simulink model "ieee_80211n"  (Simulink 7.4)
settings: Solver=ode45  StartTime=0.0  StopTime=2.076*100  RelTol=1e-3
PreLoadFcn:
  | EbNo = 1; maxNumErrs = 100; maxNumBits = 1e6;
undefined symbols (not defined in the file or in its folder): bchgenpoly
libraries: dspindex x11, dspbuff3 x6, commblkintrlv2 x4, dspxfrm3 x4, commdigbbndam3 x4, commblkcod2 x2, commsequence2 x2, commchan3 x1, commsink2 x1, commrandsrc2 x1
settings Model: Creator=nick  LastModifiedBy=nick

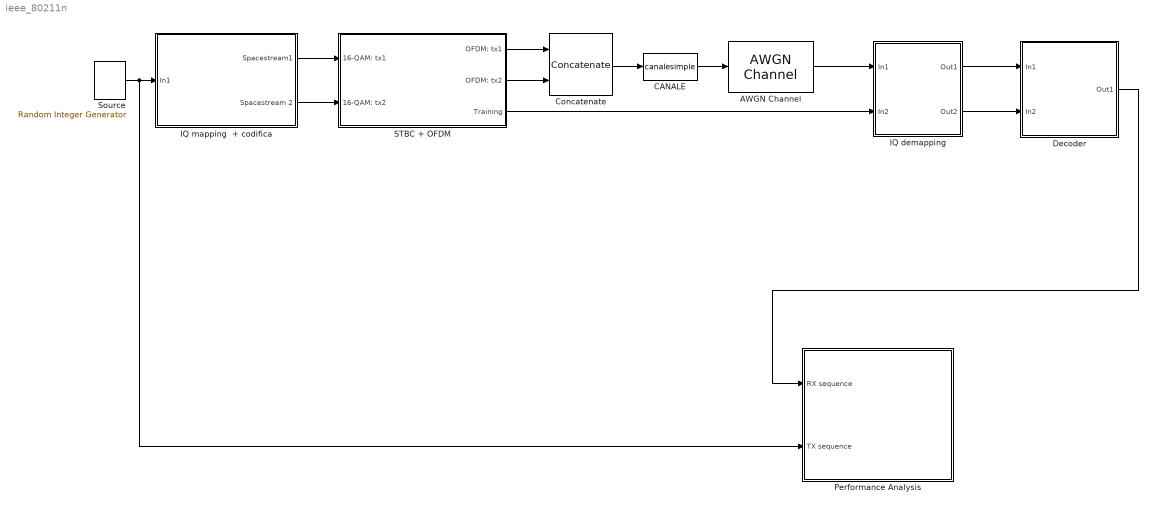
== system ieee_80211n ==
  AWGN Channel : commchan3/AWGN Channel  SystemSampleTime=-1  seed=67  noiseMode="Signal to noise ratio  (SNR)"  EbNodB=EbNo  EsNodB=10  SNRdB=SNR  bitsPerSym=264  Ps=1  Tsym=0.416  variance=1
  CANALE : MATLABFcn  MATLABFcn=canalesimple  Output1D=off
  Concatenate : Concatenate  Mode=Multidimensional array  ConcatenateDimension=2
  Decoder : Subsystem
  IQ demapping : Subsystem
  IQ mapping  + codifica : Subsystem
  Performance Analysis : Subsystem
  STBC + OFDM : Subsystem
  Source : commrandsrc2/Random Integer Generator  SystemSampleTime=-1  mul=2  seed=37  Ts=2e-3  frameBased=on  sampPerFrame=4  orient=off  outDataType=boolean
  wires:
  IQ mapping  + codifica/2(Spacestream 2) -> STBC + OFDM/2(16-QAM: tx2)
  IQ mapping  + codifica/1(Spacestream1) -> STBC + OFDM/1(16-QAM: tx1)
  Concatenate/1 -> CANALE/1
  Source/1 -> IQ mapping  + codifica/1(In1), Performance Analysis/2(TX sequence)
  STBC + OFDM/1(OFDM: tx1) -> Concatenate/1
  STBC + OFDM/2(OFDM: tx2) -> Concatenate/2
  STBC + OFDM/3(Training) -> IQ demapping/2(In2)
  CANALE/1 -> AWGN Channel/1
  IQ demapping/1(Out1) -> Decoder/1(In1)
  IQ demapping/2(Out2) -> Decoder/2(In2)
  Decoder/1(Out1) -> Performance Analysis/1(RX sequence)
  AWGN Channel/1 -> IQ demapping/1(In1)

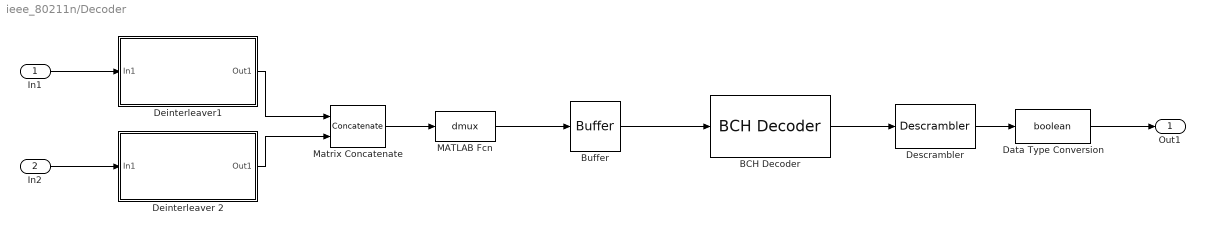
== system ieee_80211n/Decoder ==
  In1 : Inport
  In2 : Inport  Port=2
  BCH Decoder : commblkcod2/BCH Decoder  n=8  k=4  specPrimPoly=off  prPoly=de2bi(primpoly(4, 'nodisplay'), 'left-msb')  specGenPoly=off  genPoly=bchgenpoly(15,5)  specDisableGenCheck=off  specPuncture=off  punctVec=[ones(8,1); zeros(2,1)]  specErasurePort=off  showNumErr=off
  Buffer : dspbuff3/Buffer  N=8  V=0  ic=0
  Data Type Conversion : DataTypeConversion  OutDataTypeMode=boolean  OutDataType=fixdt(1, 16)  OutScaling=2^0  OutDataTypeStr=boolean
  Deinterleaver 2 : Subsystem
  Deinterleaver1 : Subsystem
  Descrambler : commsequence2/Descrambler  M=2  poly=[1 0 0 1 0 0 0 1]  ini_sta=[0 0 0 0 0 0 1]
  MATLAB Fcn : MATLABFcn  MATLABFcn=dmux  Output1D=off
  Matrix Concatenate : Concatenate  Mode=Multidimensional array  ConcatenateDimension=2
  Out1 : Outport
  wires:
  In1/1 -> Deinterleaver1/1(In1)
  In2/1 -> Deinterleaver 2/1(In1)
  Matrix Concatenate/1 -> MATLAB Fcn/1
  Deinterleaver 2/1(Out1) -> Matrix Concatenate/2
  Deinterleaver1/1(Out1) -> Matrix Concatenate/1
  BCH Decoder/1 -> Descrambler/1
  MATLAB Fcn/1 -> Buffer/1
  Data Type Conversion/1 -> Out1/1
  Descrambler/1 -> Data Type Conversion/1
  Buffer/1 -> BCH Decoder/1

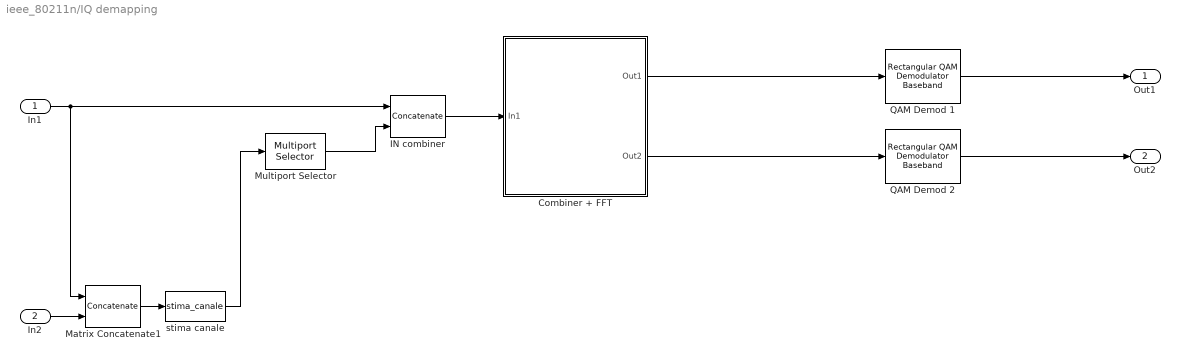
== system ieee_80211n/IQ demapping ==
  In1 : Inport
  In2 : Inport  Port=2
  Combiner + FFT : Subsystem
  IN combiner : Concatenate  Mode=Multidimensional array
  Matrix Concatenate1 : Concatenate  Mode=Multidimensional array  ConcatenateDimension=2
  Multiport Selector : dspindex/Multiport Selector  rowsOrCols=Columns  idxCellArray={ 1:2 }  idxErrMode=Clip Index
  QAM Demod 1 : commdigbbndam3/Rectangular QAM Demodulator Baseband  DialogController=commDDGCreate  DialogControllerArgs=DataTag2  M=16  PowType=Average Power  MinDist=2  AvgPow=5.25  PeakPow=1  Ph=0  Dec=Gray  Mapping=[0:15]  OutType=Bit  DecType=Hard decision  VarSource=Port  Variance=1  outDtype1=Inherit via internal rule  outDtype2=Inherit via internal rule  derotateFactorWordLen=16  denormFactorWordLen=16  prodOutWordLen=32  prodOutRoundingMode=Floor  prodOutOverflowMode=Wrap  sumWordLen=32
  QAM Demod 2 : commdigbbndam3/Rectangular QAM Demodulator Baseband  DialogController=commDDGCreate  DialogControllerArgs=DataTag3  M=16  PowType=Average Power  MinDist=2  AvgPow=5.25  PeakPow=1  Ph=0  Dec=Gray  Mapping=[0:15]  OutType=Bit  DecType=Hard decision  VarSource=Port  Variance=1  outDtype1=Inherit via internal rule  outDtype2=Inherit via internal rule  derotateFactorWordLen=16  denormFactorWordLen=16  prodOutWordLen=32  prodOutRoundingMode=Floor  prodOutOverflowMode=Wrap  sumWordLen=32
  stima canale : MATLABFcn  MATLABFcn=stima_canale  Output1D=off
  Out1 : Outport
  Out2 : Outport  Port=2
  wires:
  In1/1 -> Matrix Concatenate1/1, IN combiner/1
  Matrix Concatenate1/1 -> stima canale/1
  IN combiner/1 -> Combiner + FFT/1(In1)
  stima canale/1 -> Multiport Selector/1
  Multiport Selector/1 -> IN combiner/2
  Combiner + FFT/1(Out1) -> QAM Demod 1/1
  Combiner + FFT/2(Out2) -> QAM Demod 2/1
  QAM Demod 1/1 -> Out1/1
  QAM Demod 2/1 -> Out2/1
  In2/1 -> Matrix Concatenate1/2

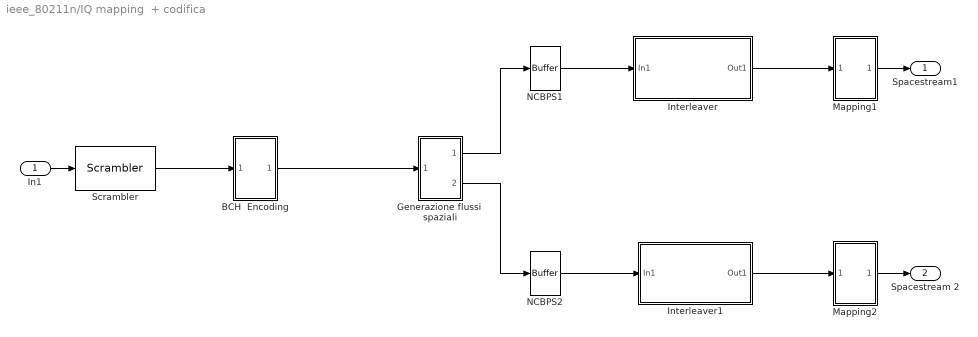
== system ieee_80211n/IQ mapping  + codifica ==
  In1 : Inport
  BCH  Encoding : Subsystem
  Generazione flussi  spaziali : Subsystem
  Interleaver : Subsystem  TreatAsAtomicUnit=on
  Interleaver1 : Subsystem  TreatAsAtomicUnit=on
  Mapping1 : Subsystem
  Mapping2 : Subsystem
  NCBPS1 : dspbuff3/Buffer  N=208  V=0  ic=0
  NCBPS2 : dspbuff3/Buffer  N=208  V=0  ic=0
  Scrambler : commsequence2/Scrambler  M=2  poly=[1 0 0 1 0 0 0 1]  ini_sta=[0 0 0 0 0 0 1]
  Spacestream1 : Outport
  Spacestream 2 : Outport  Port=2
  wires:
  Scrambler/1 -> BCH  Encoding/1(In1)
  Generazione flussi  spaziali/2(Out2) -> NCBPS2/1
  NCBPS1/1 -> Interleaver/1(In1)
  NCBPS2/1 -> Interleaver1/1(In1)
  Generazione flussi  spaziali/1(Out1) -> NCBPS1/1
  Interleaver1/1(Out1) -> Mapping2/1(In1)
  Interleaver/1(Out1) -> Mapping1/1(In1)
  Mapping1/1(Out1) -> Spacestream1/1
  Mapping2/1(Out1) -> Spacestream 2/1
  In1/1 -> Scrambler/1
  BCH  Encoding/1(Out1) -> Generazione flussi  spaziali/1(In1)

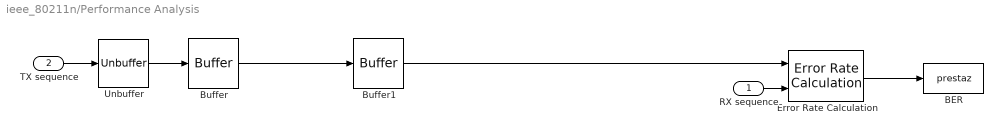
== system ieee_80211n/Performance Analysis ==
  RX sequence : Inport
  TX sequence : Inport  Port=2
  BER : ToWorkspace  VariableName=prestaz  SampleTime=-1  SaveFormat=Array
      settings: MaxDataPoints=1
  Buffer : dspbuff3/Buffer  N=208  V=0  ic=0
  Buffer1 : dspbuff3/Buffer  N=4  V=0  ic=0
  Error Rate Calculation : commsink2/Error Rate Calculation  N=0  st_delay=0  cp_mode=Entire frame  subframe=[]  PMode=Port  WsName=ErrorVec  RsMode2=off  stop=off  numErr=maxNumErrs  maxBits=maxNumBits
  Unbuffer : dspbuff3/Unbuffer  ic=0
  wires:
  Unbuffer/1 -> Buffer/1
  Buffer/1 -> Buffer1/1
  Buffer1/1 -> Error Rate Calculation/1
  Error Rate Calculation/1 -> BER/1
  TX sequence/1 -> Unbuffer/1
  RX sequence/1 -> Error Rate Calculation/2

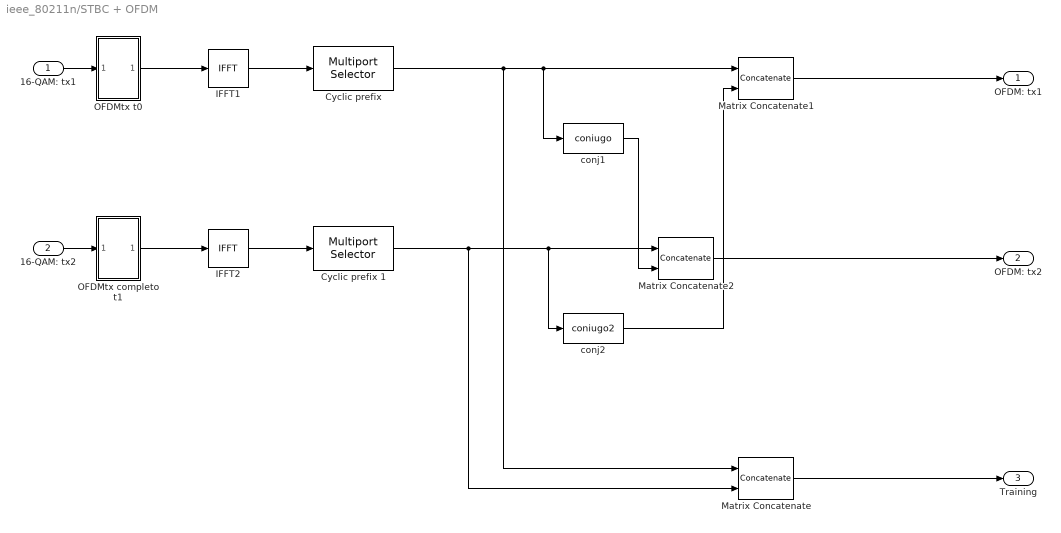
== system ieee_80211n/STBC + OFDM ==
  16-QAM: tx1 : Inport
  16-QAM: tx2 : Inport  Port=2
  Cyclic prefix : dspindex/Multiport Selector  rowsOrCols=Rows  idxCellArray={[1:64 2 1]'}  idxErrMode=Clip Index
  Cyclic prefix 1 : dspindex/Multiport Selector  rowsOrCols=Rows  idxCellArray={[1:64 2 1]'}  idxErrMode=Clip Index
  IFFT1 : dspxfrm3/IFFT  DialogController=dspDDGCreate  DialogControllerArgs=DataTag6  CompMethod=Table lookup  TableOpt=NEW  TableOptActive=Speed  BitRevOrder=off  cs_in=off  SkipNorm=on  InheritFFTLength=on  FFTLength=64  mode=Complex  outSamplingMode=Frame based  roundingMode=Floor  overflowMode=off
  IFFT2 : dspxfrm3/IFFT  DialogController=dspDDGCreate  DialogControllerArgs=DataTag7  CompMethod=Table lookup  TableOpt=NEW  TableOptActive=Speed  BitRevOrder=off  cs_in=off  SkipNorm=on  InheritFFTLength=on  FFTLength=64  mode=Complex  outSamplingMode=Frame based  roundingMode=Floor  overflowMode=off
  Matrix Concatenate : Concatenate  Mode=Multidimensional array
  Matrix Concatenate1 : Concatenate  Mode=Multidimensional array
  Matrix Concatenate2 : Concatenate  Mode=Multidimensional array
  OFDMtx completo t1 : Subsystem
  OFDMtx t0 : Subsystem
  conj1 : MATLABFcn  MATLABFcn=coniugo  Output1D=off
  conj2 : MATLABFcn  MATLABFcn=coniugo2  Output1D=off
  OFDM: tx1 : Outport  OutDataType=fixdt(1, 16)  OutScaling=2^0
  OFDM: tx2 : Outport  Port=2  OutDataType=fixdt(1, 16)  OutScaling=2^0
  Training : Outport  Port=3  OutDataType=fixdt(1, 16)  OutScaling=2^0
  wires:
  OFDMtx t0/1(Out1) -> IFFT1/1
  OFDMtx completo t1/1(Out1) -> IFFT2/1
  16-QAM: tx1/1 -> OFDMtx t0/1(In1)
  16-QAM: tx2/1 -> OFDMtx completo t1/1(In1)
  IFFT1/1 -> Cyclic prefix/1
  IFFT2/1 -> Cyclic prefix 1/1
  Cyclic prefix 1/1 -> Matrix Concatenate/2, conj2/1, Matrix Concatenate2/1
  Matrix Concatenate/1 -> Training/1
  Cyclic prefix/1 -> Matrix Concatenate1/1, conj1/1, Matrix Concatenate/1
  Matrix Concatenate1/1 -> OFDM: tx1/1
  conj1/1 -> Matrix Concatenate2/2
  Matrix Concatenate2/1 -> OFDM: tx2/1
  conj2/1 -> Matrix Concatenate1/2

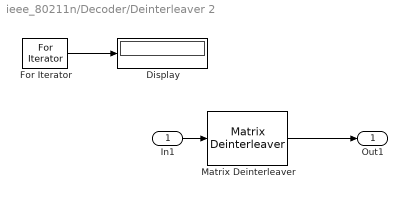
== system ieee_80211n/Decoder/Deinterleaver 2 ==
  In1 : Inport
  Display : Display
  For Iterator : ForIterator  IterationLimit=11
  Matrix Deinterleaver : commblkintrlv2/Matrix Deinterleaver  SystemSampleTime=-1  Nrows=16  Ncols=13
  Out1 : Outport  OutDataType=fixdt(1, 16)  OutScaling=2^0
  wires:
  In1/1 -> Matrix Deinterleaver/1
  Matrix Deinterleaver/1 -> Out1/1
  For Iterator/1 -> Display/1

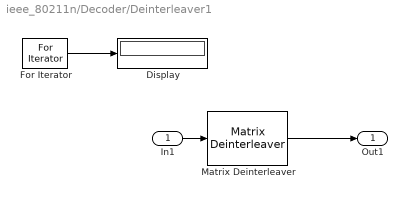
== system ieee_80211n/Decoder/Deinterleaver1 ==
  In1 : Inport
  Display : Display
  For Iterator : ForIterator  IterationLimit=11
  Matrix Deinterleaver : commblkintrlv2/Matrix Deinterleaver  SystemSampleTime=-1  Nrows=16  Ncols=13
  Out1 : Outport  OutDataType=fixdt(1, 16)  OutScaling=2^0
  wires:
  In1/1 -> Matrix Deinterleaver/1
  Matrix Deinterleaver/1 -> Out1/1
  For Iterator/1 -> Display/1

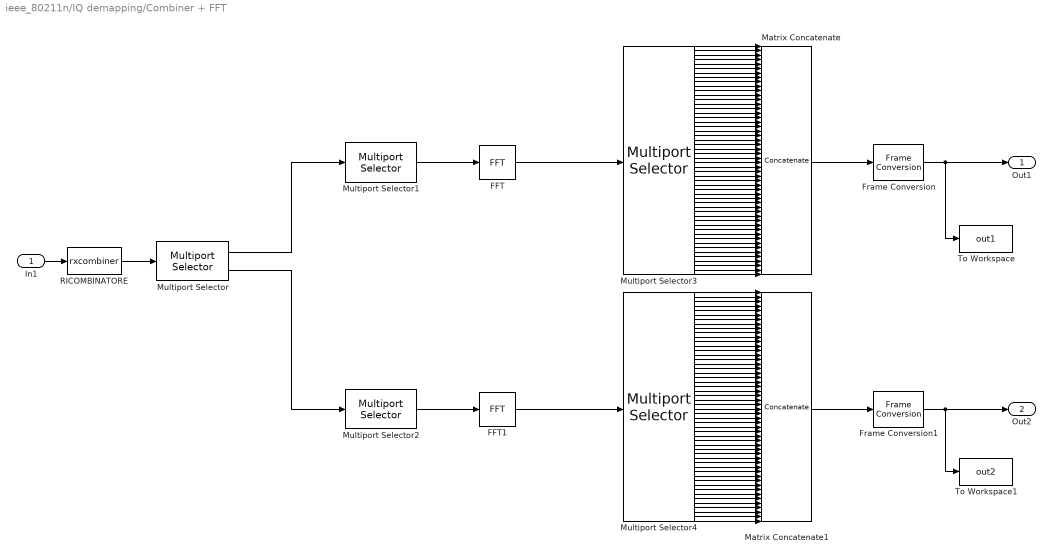
== system ieee_80211n/IQ demapping/Combiner + FFT ==
  In1 : Inport
  FFT : dspxfrm3/FFT  DialogController=dspDDGCreate  DialogControllerArgs=DataTag0  CompMethod=Table lookup  TableOpt=NEW  TableOptActive=Speed  BitRevOrder=off  InheritFFTLength=on  FFTLength=64  SkipNorm=off  roundingMode=Floor  overflowMode=off
  FFT1 : dspxfrm3/FFT  DialogController=dspDDGCreate  DialogControllerArgs=DataTag1  CompMethod=Table lookup  TableOpt=NEW  TableOptActive=Speed  BitRevOrder=off  InheritFFTLength=on  FFTLength=64  SkipNorm=off  roundingMode=Floor  overflowMode=off
  Frame Conversion : FrameConversion
  Frame Conversion1 : FrameConversion
  Matrix Concatenate : Concatenate  NumInputs=52  Mode=Multidimensional array
  Matrix Concatenate1 : Concatenate  NumInputs=52  Mode=Multidimensional array
  Multiport Selector : dspindex/Multiport Selector  rowsOrCols=Rows  idxCellArray={ [1:66],[67:132] }  idxErrMode=Clip Index
  Multiport Selector1 : dspindex/Multiport Selector  rowsOrCols=Rows  idxCellArray={ [1:64] }  idxErrMode=Clip Index
  Multiport Selector2 : dspindex/Multiport Selector  rowsOrCols=Rows  idxCellArray={ [1:64] }  idxErrMode=Clip Index
  Multiport Selector3 : dspindex/Multiport Selector  rowsOrCols=Rows  idxCellArray={2,3,4,5,6,7,9,10,11,12,13,14,15,16,17,18,19,20,21,23,24,25,26,27,28,29,37,38,39,40,41,42,44,45,46,47,48,49,50,51,52,53,54,55,56,58,59,60,61,62,63,64 }  idxErrMode=Clip Index
  Multiport Selector4 : dspindex/Multiport Selector  rowsOrCols=Rows  idxCellArray={2,3,4,5,6,7,9,10,11,12,13,14,15,16,17,18,19,20,21,23,24,25,26,27,28,29,37,38,39,40,41,42,44,45,46,47,48,49,50,51,52,53,54,55,56,58,59,60,61,62,63,64 }  idxErrMode=Clip Index
  RICOMBINATORE : MATLABFcn  MATLABFcn=rxcombiner  Output1D=off
  To Workspace : ToWorkspace  VariableName=out1  SampleTime=-1  SaveFormat=Array
  To Workspace1 : ToWorkspace  VariableName=out2  SampleTime=-1  SaveFormat=Array
  Out1 : Outport
  Out2 : Outport  Port=2
  wires:
  RICOMBINATORE/1 -> Multiport Selector/1
  Multiport Selector/1 -> Multiport Selector1/1
  Multiport Selector/2 -> Multiport Selector2/1
  Multiport Selector1/1 -> FFT/1
  Multiport Selector2/1 -> FFT1/1
  In1/1 -> RICOMBINATORE/1
  Frame Conversion/1 -> Out1/1, To Workspace/1
  FFT/1 -> Multiport Selector3/1
  Multiport Selector3/1 -> Matrix Concatenate/1
  Multiport Selector3/2 -> Matrix Concatenate/2
  Multiport Selector3/3 -> Matrix Concatenate/3
  Multiport Selector3/4 -> Matrix Concatenate/4
  Multiport Selector3/5 -> Matrix Concatenate/5
  Multiport Selector3/6 -> Matrix Concatenate/6
  Multiport Selector3/7 -> Matrix Concatenate/7
  Multiport Selector3/8 -> Matrix Concatenate/8
  Multiport Selector3/9 -> Matrix Concatenate/9
  Multiport Selector3/10 -> Matrix Concatenate/10
  Multiport Selector3/11 -> Matrix Concatenate/11
  Multiport Selector3/12 -> Matrix Concatenate/12
  Multiport Selector3/13 -> Matrix Concatenate/13
  Multiport Selector3/14 -> Matrix Concatenate/14
  Multiport Selector3/15 -> Matrix Concatenate/15
  Multiport Selector3/16 -> Matrix Concatenate/16
  Multiport Selector3/17 -> Matrix Concatenate/17
  Multiport Selector3/18 -> Matrix Concatenate/18
  Multiport Selector3/19 -> Matrix Concatenate/19
  Multiport Selector3/20 -> Matrix Concatenate/20
  Multiport Selector3/21 -> Matrix Concatenate/21
  Multiport Selector3/22 -> Matrix Concatenate/22
  Multiport Selector3/23 -> Matrix Concatenate/23
  Multiport Selector3/24 -> Matrix Concatenate/24
  Multiport Selector3/25 -> Matrix Concatenate/25
  Multiport Selector3/26 -> Matrix Concatenate/26
  Multiport Selector3/27 -> Matrix Concatenate/27
  Multiport Selector3/28 -> Matrix Concatenate/28
  Multiport Selector3/29 -> Matrix Concatenate/29
  Multiport Selector3/30 -> Matrix Concatenate/30
  Multiport Selector3/31 -> Matrix Concatenate/31
  Multiport Selector3/32 -> Matrix Concatenate/32
  Multiport Selector3/33 -> Matrix Concatenate/33
  Multiport Selector3/34 -> Matrix Concatenate/34
  Multiport Selector3/35 -> Matrix Concatenate/35
  Multiport Selector3/36 -> Matrix Concatenate/36
  Multiport Selector3/37 -> Matrix Concatenate/37
  Multiport Selector3/38 -> Matrix Concatenate/38
  Multiport Selector3/39 -> Matrix Concatenate/39
  Multiport Selector3/40 -> Matrix Concatenate/40
  Multiport Selector3/41 -> Matrix Concatenate/41
  Multiport Selector3/42 -> Matrix Concatenate/42
  Multiport Selector3/43 -> Matrix Concatenate/43
  Multiport Selector3/44 -> Matrix Concatenate/44
  Multiport Selector3/45 -> Matrix Concatenate/45
  Multiport Selector3/46 -> Matrix Concatenate/46
  Multiport Selector3/47 -> Matrix Concatenate/47
  Multiport Selector3/48 -> Matrix Concatenate/48
  Multiport Selector3/49 -> Matrix Concatenate/49
  Multiport Selector3/50 -> Matrix Concatenate/50
  Multiport Selector3/51 -> Matrix Concatenate/51
  Multiport Selector3/52 -> Matrix Concatenate/52
  Multiport Selector4/1 -> Matrix Concatenate1/1
  Multiport Selector4/2 -> Matrix Concatenate1/2
  Multiport Selector4/3 -> Matrix Concatenate1/3
  Multiport Selector4/4 -> Matrix Concatenate1/4
  Multiport Selector4/5 -> Matrix Concatenate1/5
  Multiport Selector4/6 -> Matrix Concatenate1/6
  Multiport Selector4/7 -> Matrix Concatenate1/7
  Multiport Selector4/8 -> Matrix Concatenate1/8
  Multiport Selector4/9 -> Matrix Concatenate1/9
  Multiport Selector4/10 -> Matrix Concatenate1/10
  Multiport Selector4/11 -> Matrix Concatenate1/11
  Multiport Selector4/12 -> Matrix Concatenate1/12
  Multiport Selector4/13 -> Matrix Concatenate1/13
  Multiport Selector4/14 -> Matrix Concatenate1/14
  Multiport Selector4/15 -> Matrix Concatenate1/15
  Multiport Selector4/16 -> Matrix Concatenate1/16
  Multiport Selector4/17 -> Matrix Concatenate1/17
  Multiport Selector4/18 -> Matrix Concatenate1/18
  Multiport Selector4/19 -> Matrix Concatenate1/19
  Multiport Selector4/20 -> Matrix Concatenate1/20
  Multiport Selector4/21 -> Matrix Concatenate1/21
  Multiport Selector4/22 -> Matrix Concatenate1/22
  Multiport Selector4/23 -> Matrix Concatenate1/23
  Multiport Selector4/24 -> Matrix Concatenate1/24
  Multiport Selector4/25 -> Matrix Concatenate1/25
  Multiport Selector4/26 -> Matrix Concatenate1/26
  Multiport Selector4/27 -> Matrix Concatenate1/27
  Multiport Selector4/28 -> Matrix Concatenate1/28
  Multiport Selector4/29 -> Matrix Concatenate1/29
  Multiport Selector4/30 -> Matrix Concatenate1/30
  Multiport Selector4/31 -> Matrix Concatenate1/31
  Multiport Selector4/32 -> Matrix Concatenate1/32
  Multiport Selector4/33 -> Matrix Concatenate1/33
  Multiport Selector4/34 -> Matrix Concatenate1/34
  Multiport Selector4/35 -> Matrix Concatenate1/35
  Multiport Selector4/36 -> Matrix Concatenate1/36
  Multiport Selector4/37 -> Matrix Concatenate1/37
  Multiport Selector4/38 -> Matrix Concatenate1/38
  Multiport Selector4/39 -> Matrix Concatenate1/39
  Multiport Selector4/40 -> Matrix Concatenate1/40
  Multiport Selector4/41 -> Matrix Concatenate1/41
  Multiport Selector4/42 -> Matrix Concatenate1/42
  Multiport Selector4/43 -> Matrix Concatenate1/43
  Multiport Selector4/44 -> Matrix Concatenate1/44
  Multiport Selector4/45 -> Matrix Concatenate1/45
  Multiport Selector4/46 -> Matrix Concatenate1/46
  Multiport Selector4/47 -> Matrix Concatenate1/47
  Multiport Selector4/48 -> Matrix Concatenate1/48
  Multiport Selector4/49 -> Matrix Concatenate1/49
  Multiport Selector4/50 -> Matrix Concatenate1/50
  Multiport Selector4/51 -> Matrix Concatenate1/51
  Multiport Selector4/52 -> Matrix Concatenate1/52
  Matrix Concatenate/1 -> Frame Conversion/1
  FFT1/1 -> Multiport Selector4/1
  Matrix Concatenate1/1 -> Frame Conversion1/1
  Frame Conversion1/1 -> Out2/1, To Workspace1/1

== system ieee_80211n/IQ mapping  + codifica/BCH  Encoding ==
  In1 : Inport
  BCH Encoder : commblkcod2/BCH Encoder  n=8  k=4  specPrimPoly=off  prPoly=de2bi(primpoly(4, 'nodisplay'), 'left-msb')  specGenPoly=off  genPoly=bchgenpoly(15,5)  specDisableGenCheck=off  specPuncture=off  punctVec=[ones(8,1); zeros(2,1)]
  Out1 : Outport
  wires:
  BCH Encoder/1 -> Out1/1
  In1/1 -> BCH Encoder/1

== system ieee_80211n/IQ mapping  + codifica/Generazione flussi  spaziali ==
  In1 : Inport
  spatial stream s(iss) : dspindex/Multiport Selector  rowsOrCols=Rows  idxCellArray={ 1:4, 5:8 }  idxErrMode=Clip Index
  Out1 : Outport
  Out2 : Outport  Port=2
  wires:
  spatial stream s(iss)/1 -> Out1/1
  spatial stream s(iss)/2 -> Out2/1
  In1/1 -> spatial stream s(iss)/1

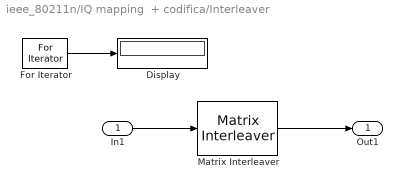
== system ieee_80211n/IQ mapping  + codifica/Interleaver ==
  In1 : Inport  OutDataType=fixdt(1, 16)  OutScaling=2^0
  Display : Display
  For Iterator : ForIterator  IterationLimit=11
  Matrix Interleaver : commblkintrlv2/Matrix Interleaver  SystemSampleTime=-1  Nrows=16  Ncols=13
  Out1 : Outport  OutDataType=fixdt(1, 16)  OutScaling=2^0
  wires:
  In1/1 -> Matrix Interleaver/1
  Matrix Interleaver/1 -> Out1/1
  For Iterator/1 -> Display/1

== system ieee_80211n/IQ mapping  + codifica/Interleaver1 ==
  In1 : Inport  OutDataType=fixdt(1, 16)  OutScaling=2^0
  Display : Display
  For Iterator : ForIterator  IterationLimit=11
  Matrix Interleaver : commblkintrlv2/Matrix Interleaver  SystemSampleTime=-1  Nrows=16  Ncols=13
  Out1 : Outport  OutDataType=fixdt(1, 16)  OutScaling=2^0
  wires:
  In1/1 -> Matrix Interleaver/1
  Matrix Interleaver/1 -> Out1/1
  For Iterator/1 -> Display/1

== system ieee_80211n/IQ mapping  + codifica/Mapping1 ==
  In1 : Inport
  mod : commdigbbndam3/Rectangular QAM Modulator Baseband  DialogController=commDDGCreate  DialogControllerArgs=DataTag4  M=16  InType=Bit  Enc=Gray  Mapping=[0:15]  PowType=Average Power  MinDist=2  AvgPow=5.25  PeakPow=1  Ph=0  outDtype=double  outWordLen=16  outUDDataType=sfix(16)  outFracLenMode=Best precision  outFracLen=15
  Out1 : Outport
  wires:
  mod/1 -> Out1/1
  In1/1 -> mod/1

== system ieee_80211n/IQ mapping  + codifica/Mapping2 ==
  In1 : Inport
  mod : commdigbbndam3/Rectangular QAM Modulator Baseband  DialogController=commDDGCreate  DialogControllerArgs=DataTag5  M=16  InType=Bit  Enc=Gray  Mapping=[0:15]  PowType=Average Power  MinDist=2  AvgPow=5.25  PeakPow=1  Ph=0  outDtype=double  outWordLen=16  outUDDataType=sfix(16)  outFracLenMode=Best precision  outFracLen=15
  Out1 : Outport
  wires:
  In1/1 -> mod/1
  mod/1 -> Out1/1

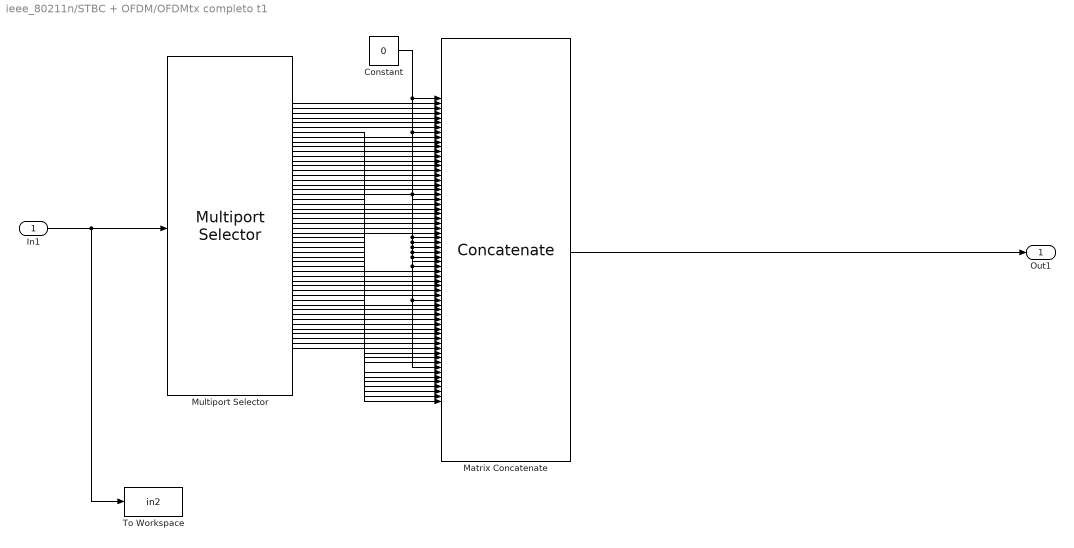
== system ieee_80211n/STBC + OFDM/OFDMtx completo t1 ==
  In1 : Inport
  Constant : Constant  Value=0  OutDataType=fixdt(1, 16)  OutScaling=2^0
  Matrix Concatenate : Concatenate  NumInputs=64  Mode=Multidimensional array
  Multiport Selector : dspindex/Multiport Selector  rowsOrCols=Rows  idxCellArray={1,2,3,4,5,6,7,8,9,10,11,12,13,14,15,16,17,18,19,20,21,22,23,24,25,26,27,28,29,30,31,32,33,34,35,36,37,38,39,40,41,42,43,44,45,46,47,48,49,50,51,52}  idxErrMode=Clip Index
  To Workspace : ToWorkspace  VariableName=in2  SampleTime=-1  SaveFormat=Array
  Out1 : Outport
  wires:
  In1/1 -> Multiport Selector/1, To Workspace/1
  Constant/1 -> Matrix Concatenate/1, Matrix Concatenate/8, Matrix Concatenate/22, Matrix Concatenate/30, Matrix Concatenate/31, Matrix Concatenate/32, Matrix Concatenate/33, Matrix Concatenate/34, Matrix Concatenate/35, Matrix Concatenate/36, Matrix Concatenate/43, Matrix Concatenate/57
  Multiport Selector/1 -> Matrix Concatenate/2
  Multiport Selector/2 -> Matrix Concatenate/3
  Multiport Selector/3 -> Matrix Concatenate/4
  Multiport Selector/4 -> Matrix Concatenate/5
  Multiport Selector/5 -> Matrix Concatenate/6
  Multiport Selector/6 -> Matrix Concatenate/7
  Multiport Selector/7 -> Matrix Concatenate/9
  Multiport Selector/8 -> Matrix Concatenate/10
  Multiport Selector/9 -> Matrix Concatenate/11
  Multiport Selector/10 -> Matrix Concatenate/12
  Multiport Selector/11 -> Matrix Concatenate/13
  Multiport Selector/12 -> Matrix Concatenate/14
  Multiport Selector/13 -> Matrix Concatenate/15
  Multiport Selector/14 -> Matrix Concatenate/16
  Multiport Selector/15 -> Matrix Concatenate/17
  Multiport Selector/16 -> Matrix Concatenate/18
  Multiport Selector/17 -> Matrix Concatenate/19
  Multiport Selector/18 -> Matrix Concatenate/20
  Multiport Selector/19 -> Matrix Concatenate/21
  Multiport Selector/20 -> Matrix Concatenate/23
  Multiport Selector/21 -> Matrix Concatenate/24
  Multiport Selector/22 -> Matrix Concatenate/25
  Multiport Selector/23 -> Matrix Concatenate/26
  Multiport Selector/24 -> Matrix Concatenate/27
  Multiport Selector/25 -> Matrix Concatenate/28
  Multiport Selector/26 -> Matrix Concatenate/29
  Multiport Selector/27 -> Matrix Concatenate/37
  Multiport Selector/28 -> Matrix Concatenate/38
  Multiport Selector/29 -> Matrix Concatenate/39
  Multiport Selector/30 -> Matrix Concatenate/40
  Multiport Selector/31 -> Matrix Concatenate/41
  Multiport Selector/32 -> Matrix Concatenate/42
  Multiport Selector/33 -> Matrix Concatenate/44
  Multiport Selector/34 -> Matrix Concatenate/45
  Multiport Selector/35 -> Matrix Concatenate/46
  Multiport Selector/36 -> Matrix Concatenate/47
  Multiport Selector/37 -> Matrix Concatenate/48
  Multiport Selector/38 -> Matrix Concatenate/49
  Multiport Selector/39 -> Matrix Concatenate/50
  Multiport Selector/40 -> Matrix Concatenate/51
  Multiport Selector/41 -> Matrix Concatenate/52
  Multiport Selector/42 -> Matrix Concatenate/53
  Multiport Selector/43 -> Matrix Concatenate/54
  Multiport Selector/44 -> Matrix Concatenate/55
  Multiport Selector/45 -> Matrix Concatenate/56
  Multiport Selector/46 -> Matrix Concatenate/58
  Multiport Selector/47 -> Matrix Concatenate/59
  Multiport Selector/48 -> Matrix Concatenate/60
  Multiport Selector/49 -> Matrix Concatenate/61
  Multiport Selector/50 -> Matrix Concatenate/62
  Multiport Selector/51 -> Matrix Concatenate/63
  Multiport Selector/52 -> Matrix Concatenate/64
  Matrix Concatenate/1 -> Out1/1

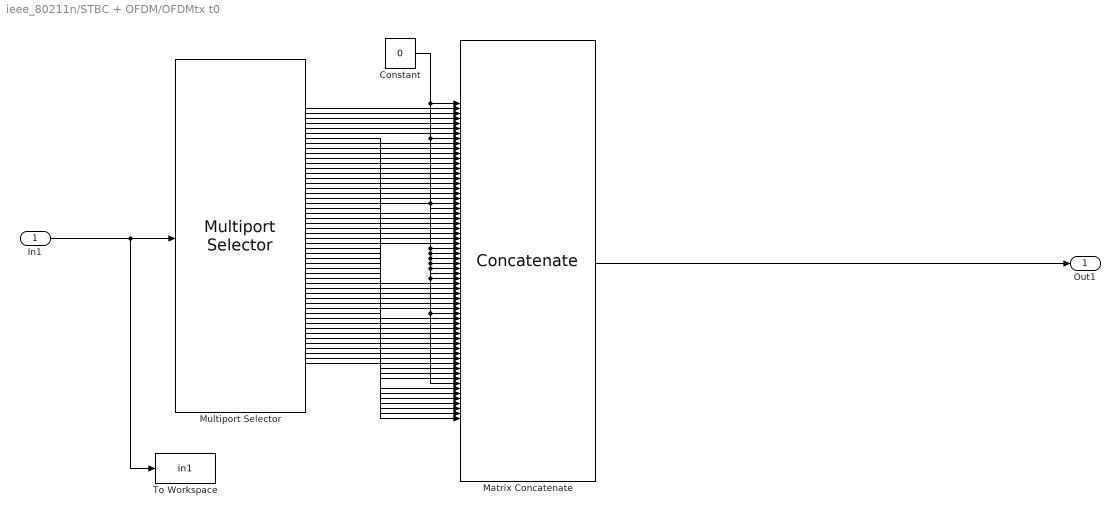
== system ieee_80211n/STBC + OFDM/OFDMtx t0 ==
  In1 : Inport
  Constant : Constant  Value=0  OutDataType=fixdt(1, 16)  OutScaling=2^0
  Matrix Concatenate : Concatenate  NumInputs=64  Mode=Multidimensional array
  Multiport Selector : dspindex/Multiport Selector  rowsOrCols=Rows  idxCellArray={1,2,3,4,5,6,7,8,9,10,11,12,13,14,15,16,17,18,19,20,21,22,23,24,25,26,27,28,29,30,31,32,33,34,35,36,37,38,39,40,41,42,43,44,45,46,47,48,49,50,51,52}  idxErrMode=Clip Index
  To Workspace : ToWorkspace  VariableName=in1  SampleTime=-1  SaveFormat=Array
  Out1 : Outport
  wires:
  Constant/1 -> Matrix Concatenate/1, Matrix Concatenate/8, Matrix Concatenate/22, Matrix Concatenate/30, Matrix Concatenate/31, Matrix Concatenate/32, Matrix Concatenate/33, Matrix Concatenate/34, Matrix Concatenate/35, Matrix Concatenate/36, Matrix Concatenate/43, Matrix Concatenate/57
  Multiport Selector/1 -> Matrix Concatenate/2
  Multiport Selector/2 -> Matrix Concatenate/3
  Multiport Selector/3 -> Matrix Concatenate/4
  Multiport Selector/4 -> Matrix Concatenate/5
  Multiport Selector/5 -> Matrix Concatenate/6
  Multiport Selector/6 -> Matrix Concatenate/7
  Multiport Selector/7 -> Matrix Concatenate/9
  Multiport Selector/8 -> Matrix Concatenate/10
  Multiport Selector/9 -> Matrix Concatenate/11
  Multiport Selector/10 -> Matrix Concatenate/12
  Multiport Selector/11 -> Matrix Concatenate/13
  Multiport Selector/12 -> Matrix Concatenate/14
  Multiport Selector/13 -> Matrix Concatenate/15
  Multiport Selector/14 -> Matrix Concatenate/16
  Multiport Selector/15 -> Matrix Concatenate/17
  Multiport Selector/16 -> Matrix Concatenate/18
  Multiport Selector/17 -> Matrix Concatenate/19
  Multiport Selector/18 -> Matrix Concatenate/20
  Multiport Selector/19 -> Matrix Concatenate/21
  Multiport Selector/20 -> Matrix Concatenate/23
  Multiport Selector/21 -> Matrix Concatenate/24
  Multiport Selector/22 -> Matrix Concatenate/25
  Multiport Selector/23 -> Matrix Concatenate/26
  Multiport Selector/24 -> Matrix Concatenate/27
  Multiport Selector/25 -> Matrix Concatenate/28
  Multiport Selector/26 -> Matrix Concatenate/29
  Multiport Selector/27 -> Matrix Concatenate/37
  Multiport Selector/28 -> Matrix Concatenate/38
  Multiport Selector/29 -> Matrix Concatenate/39
  Multiport Selector/30 -> Matrix Concatenate/40
  Multiport Selector/31 -> Matrix Concatenate/41
  Multiport Selector/32 -> Matrix Concatenate/42
  Multiport Selector/33 -> Matrix Concatenate/44
  Multiport Selector/34 -> Matrix Concatenate/45
  Multiport Selector/35 -> Matrix Concatenate/46
  Multiport Selector/36 -> Matrix Concatenate/47
  Multiport Selector/37 -> Matrix Concatenate/48
  Multiport Selector/38 -> Matrix Concatenate/49
  Multiport Selector/39 -> Matrix Concatenate/50
  Multiport Selector/40 -> Matrix Concatenate/51
  Multiport Selector/41 -> Matrix Concatenate/52
  Multiport Selector/42 -> Matrix Concatenate/53
  Multiport Selector/43 -> Matrix Concatenate/54
  Multiport Selector/44 -> Matrix Concatenate/55
  Multiport Selector/45 -> Matrix Concatenate/56
  Multiport Selector/46 -> Matrix Concatenate/58
  Multiport Selector/47 -> Matrix Concatenate/59
  Multiport Selector/48 -> Matrix Concatenate/60
  Multiport Selector/49 -> Matrix Concatenate/61
  Multiport Selector/50 -> Matrix Concatenate/62
  Multiport Selector/51 -> Matrix Concatenate/63
  Multiport Selector/52 -> Matrix Concatenate/64
  In1/1 -> Multiport Selector/1, To Workspace/1
  Matrix Concatenate/1 -> Out1/1
